simulink model "PLL_Sync_Single_Phase"  (R2019b)
settings: Solver=VariableStepAuto  StartTime=0.0  StopTime=2  FixedStep=1e-5  RelTol=1e-3
libraries: powerlib x15, powerlib_meascontrol x2, dspswit3 x1, simulink x1
settings Model: Creator=cy5924je  LastModifiedBy=samue
settings DataIOCC: ReturnWorkspaceOutputs=off
settings DebuggingCC: ArithmeticOperatorsInVariantConditions=warning
settings SFSimCC: SimUseLocalCustomCode=off  CustomCodeUndefinedFunction=UseInterfaceOnly
settings RTWCC: RTWUseLocalCustomCode=off

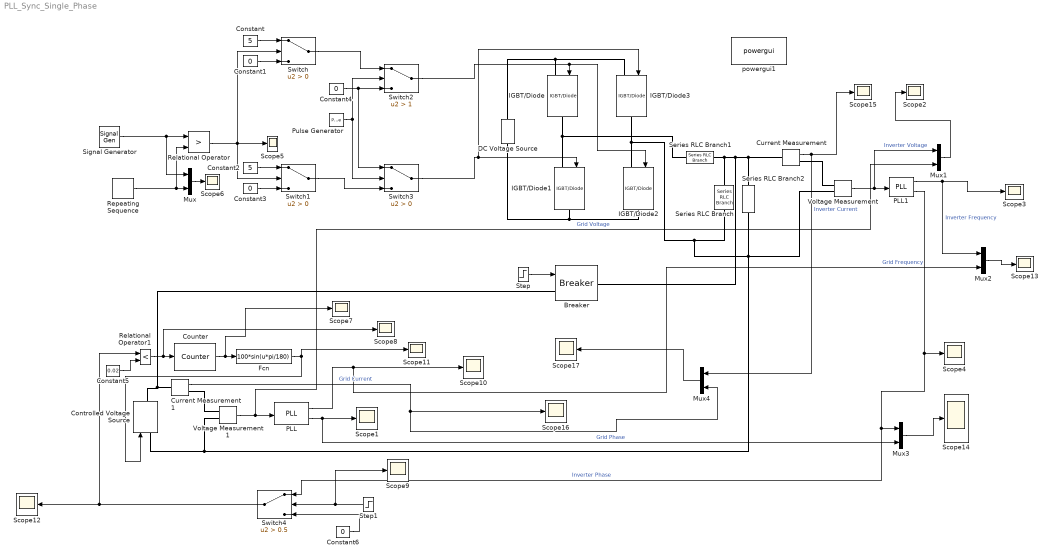
== system PLL_Sync_Single_Phase ==
  Breaker : powerlib/Elements/Breaker  InitialState=0  SwitchingTimes="[1/60  5/60]"  External=on  BreakerResistance=0.01  SnubberResistance=1e6  SnubberCapacitance=inf  Measurements=None  MoreParameters=on  NoBreakLoop=off
      settings: SourceProductName=Simscape Electrical
  Constant : Constant  Value=5
  Constant{1,3..4,6} (4 alike) : Constant  Value=0
  Constant2 : Constant  Value=5
  Constant5 : Constant  Value=0.02
  Controlled Voltage Source : powerlib/Electrical Sources/Controlled Voltage Source  Initialize=on  Source_Type=AC  Amplitude=0  Phase=0  Frequency=60  Measurements=None
      settings: SourceProductName=Simscape Electrical
  Counter : dspswit3/Counter  Direction=Up  CountEvent=Free running  CounterSize=User defined  MaxCount=360  InitialCount=0  Output=Count  HitValue=32  ResetInput=on  SamplesPerFrame=1  Ts=5e-5  CntDtype=double  HitDtype=Logical
  Current Measurement : powerlib/Measurements/Current Measurement  PhasorSimulation=off  OutputType=Complex  PSBequivalent=0
      settings: SourceProductName=Simscape Electrical
  Current Measurement1 : powerlib/Measurements/Current Measurement  PhasorSimulation=off  OutputType=Complex  PSBequivalent=0
      settings: SourceProductName=Simscape Electrical
  DC Voltage Source : powerlib/Electrical Sources/DC Voltage Source  Amplitude=100  Measurements=None
      settings: SourceProductName=Simscape Electrical
  Fcn : Fcn  Expr=100*sin(u*pi/180)
  IGBT/Diode{,1..3} (4 alike) : powerlib/Power Electronics/IGBT//Diode  Ron=1e-3  Rs=1e5  Cs=inf  Measurements=off
      settings: SourceProductName=Simscape Electrical
  Mux{,1..4} (5 alike) : Mux  Inputs=2
  PLL : powerlib_meascontrol/PLL/PLL  Fmin=45  Par_Init=[0, 60]  ParK=[180, 3200, 1]  TcD=1e-4  MaxRateChangeFreq=12  FilterCutOffFreq=25  Ts=0  AGC=on
      settings: SourceProductName=Simscape Electrical  SourceProductBaseCode=PS
  PLL1 : powerlib_meascontrol/PLL/PLL  Fmin=45  Par_Init=[0, 60]  ParK=[180, 3200, 1]  TcD=1e-4  MaxRateChangeFreq=12  FilterCutOffFreq=25  Ts=5e-5  AGC=on
      settings: SourceProductName=Simscape Electrical  SourceProductBaseCode=PS
  Pulse Generator : DiscretePulseGenerator  PulseType=Time based  Amplitude=2  Period=1/60  PulseWidth=50
  Relational Operator : RelationalOperator  Operator=>  OutDataTypeStr=boolean  RndMeth=Simplest
  Relational Operator1 : RelationalOperator  Operator=<  OutDataTypeStr=boolean  RndMeth=Simplest
  Repeating Sequence : simulink/Sources/Repeating Sequence  rep_seq_t=[0 1/4800 1/2400]  rep_seq_y=[0 100 0]
  Scope{1..17} (17 alike) : Scope
  Series RLC Branch : powerlib/Elements/Series RLC Branch  LConnTagsString=__new0  RConnTagsString=__new0  BranchType=C  Resistance=0  Inductance=1e-3  SetiL0=off  InitialCurrent=0  Capacitance=5e-6  Setx0=off  InitialVoltage=0  Measurements=None
      settings: SourceProductName=Simscape Electrical
  Series RLC Branch1 : powerlib/Elements/Series RLC Branch  LConnTagsString=__new0  RConnTagsString=__new0  BranchType=L  Resistance=10  Inductance=5e-3  SetiL0=off  InitialCurrent=0  Capacitance=0.1e-7  Setx0=off  InitialVoltage=0  Measurements=None
      settings: SourceProductName=Simscape Electrical
  Series RLC Branch2 : powerlib/Elements/Series RLC Branch  LConnTagsString=__new0  RConnTagsString=__new0  BranchType=R  Resistance=100  Inductance=1e-3  SetiL0=off  InitialCurrent=0  Capacitance=0.1e-7  Setx0=off  InitialVoltage=0  Measurements=None
      settings: SourceProductName=Simscape Electrical
  Signal Generator : SignalGenerator  Amplitude=100  Frequency=60
  Step : Step  Time=0.1  SampleTime=0
  Step1 : Step  Time=0.06  SampleTime=0
  Switch : Switch  Criteria=u2 > Threshold  RndMeth=Zero
  Switch1 : Switch  Criteria=u2 > Threshold
  Switch2 : Switch  Criteria=u2 > Threshold  Threshold=1  RndMeth=Zero
  Switch3 : Switch  Criteria=u2 > Threshold  RndMeth=Zero
  Switch4 : Switch  Criteria=u2 > Threshold  Threshold=0.5  RndMeth=Zero
  Voltage Measurement : powerlib/Measurements/Voltage Measurement  PhasorSimulation=off  OutputType=Complex  PSBequivalent=0
      settings: SourceProductName=Simscape Electrical
  Voltage Measurement1 : powerlib/Measurements/Voltage Measurement  PhasorSimulation=off  OutputType=Complex  PSBequivalent=0
      settings: SourceProductName=Simscape Electrical
  powergui1 : powerlib/powergui  Priority=1  SimulationMode=Discrete  SampleTime=50e-6  frequency=60  Iterations=50  frequencyindice=60  Pbase=100e6  ErrMax=1e-4  UnitsV=kV  UnitsW=MW  buscounter=0  FunctionMessages=off  echomessages=off  EnableUseOfTLC=off  CurrentSourceSwitches=off  DisableSnubberDevices=off  DisableRonSwitches=off  DisableVfSwitches=off  DisplayEquations=off  AutomaticDiscreteSolvers=off  SolverType=Tustin/Backward Euler (TBE)  Interpol=off  ExternalGateDelay=off  methode=off  Ts=100  x0status=blocks  SPID=off  SwTol=0  HookPort=off  NonlinearTolerance=1e-4  nMaxIteration=100  ContinueOnMaxIteration=off  RestoreLinks=warning  ResistiveCurrentMeasurement=off  Frange=[0:2:500]  Ylog=off  Xlog=on  ShowGrid=off  save=off  variable=ZData  structure=0  ZoomFFT=off  StartTime=0.0  cycles=1  DisplayStyle=1  fundamental=60  FreqAxis=off  MaxFrequency=1000  frequencyindicesteady=1  RmsSteady=1  display=off
      settings: SourceProductName=Simscape Electrical
  wires:
  Relational Operator/1 -> Switch1/2, Switch/2, Scope5/1
  Constant/1 -> Switch/1
  Constant1/1 -> Switch/3
  Voltage Measurement/1 -> Mux1/1, PLL1/1  "Inverter Voltage"
  Constant2/1 -> Switch1/1
  Constant3/1 -> Switch1/3
  Repeating Sequence/1 -> Relational Operator/2, Mux/2
  Mux/1 -> Scope6/1
  Pulse Generator/1 -> Switch3/2, Switch2/2
  Switch/1 -> Switch2/1
  Switch1/1 -> Switch3/3
  Constant4/1 -> Switch2/3, Switch3/1
  Switch2/1 -> IGBT/Diode2/1, IGBT/Diode/1
  Switch3/1 -> IGBT/Diode3/1, IGBT/Diode1/1
  PLL/2 -> Mux3/2, Scope1/1  "Grid Phase"
  Step/1 -> Breaker/1
  Voltage Measurement1/1 -> Mux1/2, PLL/1  "Grid Voltage"
  Counter/1 -> Scope7/1, Fcn/1
  Fcn/1 -> Scope11/1, Controlled Voltage Source/1
  PLL1/2 -> Mux3/1, Switch4/1, Scope4/1  "Inverter Phase"
  Relational Operator1/1 -> Scope8/1, Counter/1
  Constant5/1 -> Relational Operator1/2
  Step1/1 -> Scope9/1, Switch4/2
  Constant6/1 -> Switch4/3
  Switch4/1 -> Relational Operator1/1, Scope12/1
  Mux1/1 -> Scope2/1
  PLL1/1 -> Mux2/1, Scope3/1  "Inverter Frequency"
  PLL/1 -> Mux2/2, Scope10/1  "Grid Frequency"
  Mux2/1 -> Scope13/1
  Mux3/1 -> Scope14/1
  Current Measurement/1 -> Mux4/1, Scope15/1  "Inverter Current"
  Current Measurement1/1 -> Mux4/2, Scope16/1  "Grid Current"
  Mux4/1 -> Scope17/1
  Signal Generator/1 -> Mux/1, Relational Operator/1
  connections:
  DC Voltage Source/RConn1 -- IGBT/Diode3/LConn1 -- IGBT/Diode/LConn1
  IGBT/Diode1/RConn1 -- DC Voltage Source/LConn1 -- IGBT/Diode2/RConn1
  IGBT/Diode/RConn1 -- IGBT/Diode1/LConn1 -- Series RLC Branch1/RConn1
  IGBT/Diode3/RConn1 -- Series RLC Branch/RConn1 -- Voltage Measurement/LConn2 -- Controlled Voltage Source/LConn1 -- Voltage Measurement1/LConn2 -- Series RLC Branch2/LConn1 -- IGBT/Diode2/LConn1
  Series RLC Branch1/LConn1 -- Series RLC Branch/LConn1 -- Breaker/RConn1 -- Series RLC Branch2/RConn1 -- Current Measurement/LConn1
  Current Measurement/RConn1 -- Voltage Measurement/LConn1
  Current Measurement1/LConn1 -- Controlled Voltage Source/RConn1 -- Breaker/LConn1
  Current Measurement1/RConn1 -- Voltage Measurement1/LConn1
